simulink model "Sepic_Converter_PV_Mean_C1"  (R2016b)
settings: Solver=VariableStepAuto  StartTime=0.0  StopTime=5  RelTol=1e-3  EnableMultiTasking=on
libraries: powerlib x25, powerlib_meascontrol x6, dspstat3 x3, re_lib x1
settings Model: Creator=Rangga  LastModifiedBy=Rangga Putra
settings OptimizationCC: LifeSpan=inf
settings DebuggingCC: SFUnexpectedBacktrackingDiag=warning  SFNoUnconditionalDefaultTransitionDiag=warning  SFExecutionAtInitializationDiag=none
settings GRTTargetCC: TargetLangStandard=C89/C90 (ANSI)  GeneratePreprocessorConditionals=Disable all
settings ConfigComp: CovMetricSettings=dw  CovHtmlReporting=on  CovSaveCumulativeToWorkspaceVar=on  CovSaveSingleToWorkspaceVar=on  CovExternalEMLEnable=off

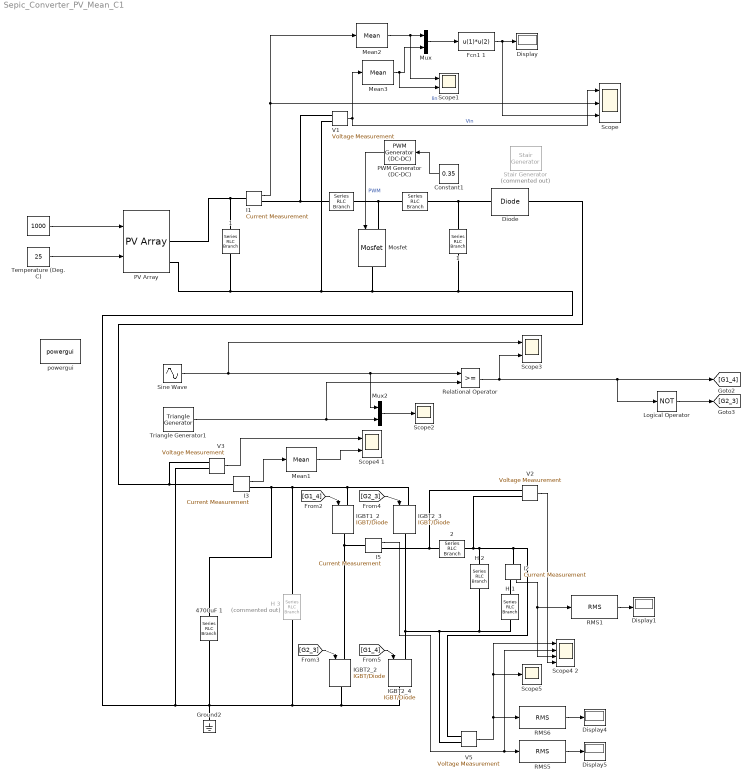
== system Sepic_Converter_PV_Mean_C1 ==
  " " : Constant  Value=1000
  " " : powerlib/Elements/Series RLC Branch  LConnTagsString=__new0  RConnTagsString=__new0  BranchType=L  Resistance=2  Inductance=2.5e-3  SetiL0=off  InitialCurrent=0  Capacitance=[]  Setx0=off  InitialVoltage=0  Measurements=None
  " " : powerlib/Elements/Series RLC Branch  LConnTagsString=__new0  RConnTagsString=__new0  BranchType=C  Resistance=3000e-6  Inductance=2e-3  SetiL0=off  InitialCurrent=0  Capacitance=0.001  Setx0=off  InitialVoltage=10  Measurements=None
  " 1" : powerlib/Elements/Series RLC Branch  LConnTagsString=__new0  RConnTagsString=__new0  BranchType=C  Resistance=3000e-6  Inductance=2e-3  SetiL0=off  InitialCurrent=0  Capacitance=0.001  Setx0=off  InitialVoltage=10  Measurements=None
  " 1" : powerlib/Elements/Series RLC Branch  LConnTagsString=__new0  RConnTagsString=__new0  BranchType=L  Resistance=2  Inductance=0.1e-3  SetiL0=off  InitialCurrent=0  Capacitance=[]  Setx0=off  InitialVoltage=0  Measurements=None
  " 2" : powerlib/Elements/Series RLC Branch  LConnTagsString=__new0  RConnTagsString=__new0  BranchType=L  Resistance=3  Inductance=1500e-6  SetiL0=off  InitialCurrent=0  Capacitance=[]  Setx0=off  InitialVoltage=0  Measurements=None
  4700uF 1 : powerlib/Elements/Series RLC Branch  LConnTagsString=__new0  RConnTagsString=__new0  BranchType=C  Resistance=3  Inductance=2e-3  SetiL0=off  InitialCurrent=0  Capacitance=4700e-6  Setx0=off  InitialVoltage=0  Measurements=None
  Constant1 : Constant  Value=0.35
  Diode : powerlib/Power Electronics/Diode  Ron=0.0001  Lon=0  Vf=0.8  IC=0  UseSnubber=off  Rs=0  Cs=0  Measurements=off
  Display{,1,4..5} (4 alike) : Display
      Display4 settings: Decimation=3
  Fcn1 1 : Fcn  Expr=u(1)*u(2)
  Ground2 : powerlib/Elements/Ground  LConnTagsString=a
  H 1 : powerlib/Elements/Series RLC Branch  LConnTagsString=__new0  RConnTagsString=__new0  BranchType=RL  Resistance=2  Inductance=100e-6  SetiL0=off  InitialCurrent=0  Capacitance=1000e-6  Setx0=off  InitialVoltage=0  Measurements=None
  H 2 : powerlib/Elements/Series RLC Branch  LConnTagsString=__new0  RConnTagsString=__new0  BranchType=C  Resistance=1  Inductance=2e-3  SetiL0=off  InitialCurrent=0  Capacitance=10e-6  Setx0=off  InitialVoltage=0  Measurements=None
  H 3 : powerlib/Elements/Series RLC Branch  Commented=on  LConnTagsString=__new0  RConnTagsString=__new0  BranchType=RL  Resistance=2  Inductance=100e-6  SetiL0=off  InitialCurrent=0  Capacitance=1000e-6  Setx0=off  InitialVoltage=0  Measurements=None
  I{1..3,5} (4 alike) : powerlib/Measurements/Current Measurement  Tag=PoWeRsYsTeMmEaSuReMeNt  PhasorSimulation=off  OutputType=Magnitude  PSBequivalent=0
  IGBT1_2 : powerlib/Power Electronics/IGBT//Diode  Ron=1e-3  Rs=1e5  Cs=inf  Measurements=off
  IGBT2_2 : powerlib/Power Electronics/IGBT//Diode  Ron=1e-3  Rs=1e5  Cs=inf  Measurements=off
  IGBT2_3 : powerlib/Power Electronics/IGBT//Diode  Ron=1e-3  Rs=1e5  Cs=inf  Measurements=off
  IGBT2_4 : powerlib/Power Electronics/IGBT//Diode  Ron=1e-3  Rs=1e5  Cs=inf  Measurements=off
  Logical Operator : Logic  Operator=NOT  AllPortsSameDT=off  OutDataTypeStr=boolean
  Mean1 : powerlib_meascontrol/Measurements/Mean  Freq=60  Vinit=0  Ts=0
  Mean2 : powerlib_meascontrol/Measurements/Mean  Freq=60  Vinit=0  Ts=0
  Mean3 : powerlib_meascontrol/Measurements/Mean  Freq=60  Vinit=0  Ts=0
  Mosfet : powerlib/Power Electronics/Mosfet  Ron=0.01  Lon=0  Rd=0.01  Vfd=0  IC=0  Rs=1e5  Cs=inf  Measurements=off
  Mux : Mux  Inputs=2
  Mux2 : Mux  Inputs=2
  PV Array : re_lib/Solar/PV Array  Npar=1  Nser=1  PlotType=one module @ 25 deg.C & specified irradiances  S_vec=1000  Temp_C_vec=[ 45 25 100 ]  ModuleName=User-defined  PlotWhenSelected=off  Pm=99.981  Ncell=36  Voc=22.5  Isc=5.75  Vm=18.9  Im=5.29  beta_Voc_pc=-0.35  alpha_Isc_pc=0.06  beta_Voc=-0.07875  alpha_Isc=0.00345  IL=5.7591  I0=1.3543e-10  nI=0.99573  Rsh=93.7325  Rs=0.14801  BAL=on  Tc=1e-6  Tfilter=5e-5
      settings: AttributesFormatString=|
      | %<ModuleName>
      | %<Nser>-module string
      | %<Npar> parallel strings
  "PWM Generator (DC-DC) " : powerlib_meascontrol/Pulse & Signal Generators/PWM Generator (DC-DC)  Fsw=5000  Ts=0
  RMS1 : dspstat3/RMS  run=on  directionMode=Each column  dimension=1  InputProcessing=Columns as channels (frame based)  reset_popup=None
  RMS5 : dspstat3/RMS  run=on  directionMode=Each column  dimension=1  InputProcessing=Columns as channels (frame based)  reset_popup=None
  RMS6 : dspstat3/RMS  run=on  directionMode=Each column  dimension=1  InputProcessing=Columns as channels (frame based)  reset_popup=None
  Relational Operator : RelationalOperator  OutDataTypeStr=boolean  RndMeth=Nearest
  Scope : Scope  NumInputPorts=3
  Scope1 : Scope  NumInputPorts=2
  Scope2 : Scope
  Scope3 : Scope  NumInputPorts=2
  Scope4 1 : Scope  NumInputPorts=2
  Scope4 2 : Scope  NumInputPorts=4
  Scope5 : Scope
  Sine Wave : Sin  Amplitude=0.5  Frequency=2*pi*60  SampleTime=0
  Stair Generator : powerlib_meascontrol/Pulse & Signal Generators/Stair Generator  Commented=on  t=[0, 1, 2, 3, 4, 5, 6, 7, 8]  e=[0.1, 0.2, 0.3, 0.4, 0.5, 0.6, 0.7, 0.8, 0.9]  Ts=0
  Temperature (Deg. C) : Constant  Value=25
  Triangle Generator1 : powerlib_meascontrol/Pulse & Signal Generators/Triangle Generator  Freq=10000  Phase=0  Ts=0
  V{1..3,5} (4 alike) : powerlib/Measurements/Voltage Measurement  Tag=PoWeRsYsTeMmEaSuReMeNt  PhasorSimulation=off  OutputType=Magnitude  PSBequivalent=0
  powergui : powerlib/powergui  Priority=1  SimulationMode=Discrete  SolverType=Tustin/Backward Euler (TBE)  SampleTime=1e-6  frequency=60  SPID=off  DisableSnubberDevices=off  DisableRonSwitches=off  DisableVfSwitches=off  SwTol=0  DisplayEquations=off  Interpol=off  ExternalGateDelay=off  methode=off  Ts=10  FunctionMessages=off  echomessages=off  HookPort=off  EnableUseOfTLC=off  x0status=blocks  frequencyindice=0  Pbase=100e6  ErrMax=1e-4  Iterations=50  UnitsV=kV  UnitsW=MW  buscounter=0  RestoreLinks=warning  ResistiveCurrentMeasurement=off  Frange=[0:2:500]  Ylog=off  Xlog=on  ShowGrid=off  save=off  variable=ZData  structure=0  ZoomFFT=off  StartTime=0.0  cycles=1  DisplayStyle=1  fundamental=60  FreqAxis=off  MaxFrequency=1000  frequencyindicesteady=1  RmsSteady=1  display=off
  wires:
  "PWM Generator (DC-DC) "/1 -> Mosfet/1  "PWM"
  V1/1 -> Mean3/1, Scope/1  "Vin"
  I1/1 -> Mean2/1, Scope/2  "Iin"
  Fcn1 1/1 -> Scope/3, Display/1
  Mux/1 -> Fcn1 1/1
  Mean2/1 -> Scope1/1, Mux/1
  Mean3/1 -> Scope1/2, Mux/2
  " "/1 -> PV Array/1
  Temperature (Deg. C)/1 -> PV Array/2
  [G1_4] -> IGBT1_2/1
  [G2_3] -> IGBT2_2/1
  [G2_3] -> IGBT2_3/1
  [G1_4] -> IGBT2_4/1
  Sine Wave/1 -> Scope3/1, Mux2/1, Relational Operator/1
  Relational Operator/1 -> Scope3/2, Logical Operator/1, [G1_4]
  Logical Operator/1 -> [G2_3]
  Triangle Generator1/1 -> Mux2/2, Relational Operator/2
  Mux2/1 -> Scope2/1
  I5/1 -> Scope4 2/2, RMS5/1
  V5/1 -> Scope4 2/1, Scope5/1, RMS6/1
  V3/1 -> Scope4 1/1
  I3/1 -> Mean1/1
  RMS6/1 -> Display4/1
  RMS5/1 -> Display5/1
  V2/1 -> Scope4 2/4
  I2/1 -> RMS1/1, Scope4 2/3
  RMS1/1 -> Display1/1
  Constant1/1 -> "PWM Generator (DC-DC) "/1
  Mean1/1 -> Scope4 1/2
  connections:
  " "/RConn1 -- I1/RConn1 -- V1/LConn1
  IGBT2_2/RConn1 -- H 3/RConn1 -- Ground2/LConn1 -- " 1"/LConn1 -- Mosfet/RConn1 -- V1/LConn2 -- PV Array/RConn2 -- " 1"/RConn1 -- V3/LConn2 -- 4700uF 1/RConn1 -- IGBT2_4/RConn1
  " "/LConn1 -- " 1"/RConn1 -- Diode/LConn1
  V3/LConn1 -- I3/LConn1 -- Diode/RConn1
  " "/LConn1 -- Mosfet/LConn1 -- " "/RConn1
  PV Array/RConn1 -- " 1"/LConn1 -- I1/LConn1
  IGBT2_3/LConn1 -- H 3/LConn1 -- 4700uF 1/LConn1 -- I3/RConn1 -- IGBT1_2/LConn1
  IGBT2_2/LConn1 -- IGBT1_2/RConn1 -- I5/LConn1
  IGBT2_4/LConn1 -- IGBT2_3/RConn1 -- H 2/RConn1 -- H 1/RConn1 -- V5/LConn2
  I5/RConn1 -- V2/LConn1 -- " 2"/RConn1
  V5/LConn1 -- I2/LConn1 -- V2/LConn2 -- " 2"/LConn1 -- H 2/LConn1
  I2/RConn1 -- H 1/LConn1
